simulink model "ProbeFailureDetector"  (R2025a)
settings: Solver=ode23tb  StartTime=0.0  StopTime=1000  MaxStep=0.1  RelTol=1e-3
model workspace (MAT data in the model file):
  max_probe_height = 15.44
undefined symbols (not defined in the file): FAILURE_OPEN_THRESH, FAILURE_RATE_THRESH, FAILURE_SHORT_MARGIN
libraries: simulink x2
settings Model: DataDictionary=FuelGaugingData.sldd  Creator=mkelley  LastModifiedBy=mkelley

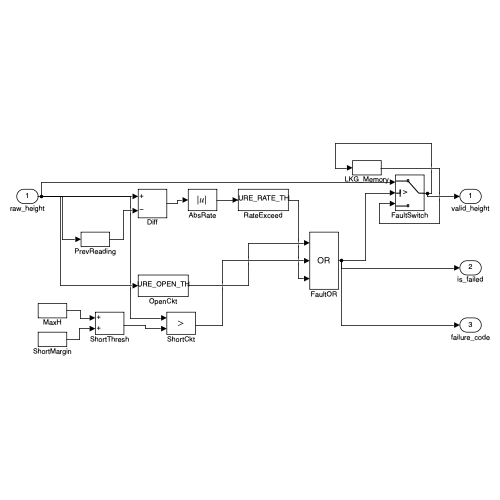
[thumbnail: Simulink's stored preview of the top-level diagram]
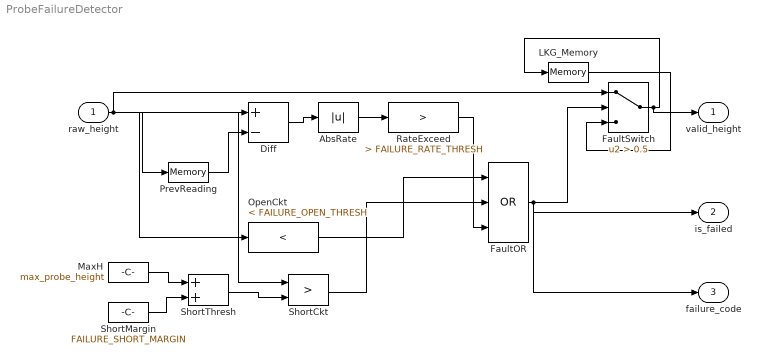
== system ProbeFailureDetector ==
  raw_height : Inport
  AbsRate : Abs  SaturateOnIntegerOverflow=off
  Diff : Sum  Inputs=+-
  FaultOR : Logic  Operator=OR  Inputs=3  AllPortsSameDT=off  OutDataTypeStr=boolean
  FaultSwitch : Switch  Criteria=u2 > Threshold  Threshold=0.5  SaturateOnIntegerOverflow=off  InputSameDT=off
  LKG_Memory : Memory
  MaxH : Constant  Value=max_probe_height
  OpenCkt : simulink/Logic and Bit Operations/Compare To Constant  relop=<  const=FAILURE_OPEN_THRESH  OutDataTypeStr=boolean
  PrevReading : Memory
  RateExceed : simulink/Logic and Bit Operations/Compare To Constant  relop=>  const=FAILURE_RATE_THRESH  OutDataTypeStr=boolean
  ShortCkt : RelationalOperator  Operator=>  OutDataTypeStr=boolean  RndMeth=Simplest  InputSameDT=off
  ShortMargin : Constant  Value=FAILURE_SHORT_MARGIN
  ShortThresh : Sum
  valid_height : Outport
  is_failed : Outport  Port=2
  failure_code : Outport  Port=3
  wires:
  raw_height/1 -> PrevReading/1, Diff/1, OpenCkt/1, ShortCkt/1, FaultSwitch/1
  PrevReading/1 -> Diff/2
  Diff/1 -> AbsRate/1
  AbsRate/1 -> RateExceed/1
  MaxH/1 -> ShortThresh/1
  ShortMargin/1 -> ShortThresh/2
  ShortThresh/1 -> ShortCkt/2
  OpenCkt/1 -> FaultOR/1
  ShortCkt/1 -> FaultOR/2
  RateExceed/1 -> FaultOR/3
  FaultOR/1 -> FaultSwitch/2, is_failed/1, failure_code/1
  LKG_Memory/1 -> FaultSwitch/3
  FaultSwitch/1 -> LKG_Memory/1, valid_height/1
